simulink model "massspringtask"  (R2022b)
settings: Solver=VariableStepAuto  StartTime=0.0  StopTime=10.0  RelTol=1e-3
settings Model: Creator=brbar  LastModifiedBy=brbar

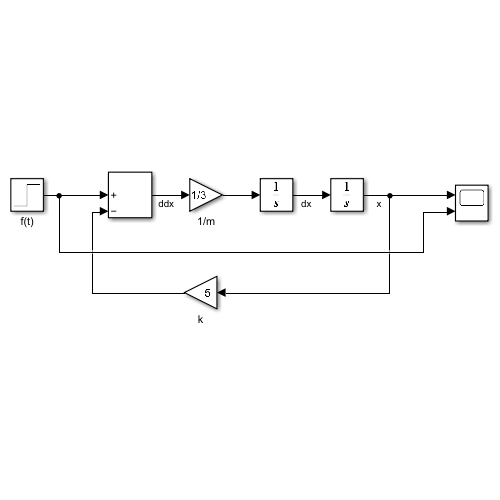
[thumbnail: Simulink's stored preview of the top-level diagram]
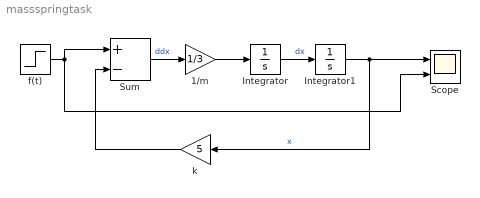
== system massspringtask ==
  1/m : Gain  Gain=1/3
  Integrator : Integrator
  Integrator1 : Integrator
  Scope : Scope  NumInputPorts=2
  Sum : Sum  Inputs=|+-
  f(t) : Step  SampleTime=0
  k : Gain  Gain=5
  wires:
  Integrator/1 -> Integrator1/1  "dx"
  Integrator1/1 -> Scope/1, k/1  "x"
  k/1 -> Sum/2
  f(t)/1 -> Scope/2, Sum/1
  Sum/1 -> 1/m/1  "ddx"
  1/m/1 -> Integrator/1
